simulink model "GFLIB_ControllerPIr_BAM_F32"  (Simulink 7.3)
settings: Solver=ode45  StartTime=0.0  StopTime=10.0  RelTol=1e-3
undefined symbols (not defined in the file): f32CC1, f32CC2, u16NShift
settings Model: Creator=RE004C  LastModifiedBy=RE004C
settings HardwareCC: ProdIntDivRoundTo=Zero  ProdEndianess=BigEndian  ProdHWDeviceType=Freescale->32-bit PowerPC

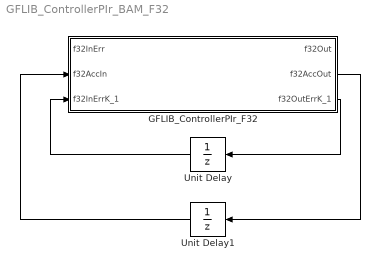
== system GFLIB_ControllerPIr_BAM_F32 ==
  GFLIB_ControllerPIr_F32 : Subsystem  mask(GFLIB_ControllerPIr_F32){f32CC1=f32CC1, f32CC2=f32CC2, u16NShift=u16NShift}
      mask help: Bit accurate model of reccurent form PI controller. All parameters as well as input and output are 32-bit integers except for u16NShift parameter which is 16-bit unsigned integer.
      mask init:
      | pos = get_param(gcb, 'Position');width = pos(3) - pos(1); height = pos(4) - pos(2);tX=width/2;tY=height*0.9;
      mask Display:
      | color('black');
      | port_label('input',1,'f32InErr');
      | port_label('input',2,'f32AccIn');
      | port_label('input',3,'f32InErrK_1');
      | port_label('output',1,'f32Out');
      | port_label('output',2,'f32AccOut');
      | port_label('output',3,'f32OutErrK_1');
      | color('black');
      | disp('GFLIB_ControllerPIr_F32');
      | color('blue');
      | text(tX,tY, 'BAM', 'horizontalAlignment', 'center');
  Unit Delay : UnitDelay  SampleTime=-1
  Unit Delay1 : UnitDelay  SampleTime=-1
  wires:
  GFLIB_ControllerPIr_F32/3(f32OutErrK_1) -> Unit Delay/1
  Unit Delay/1 -> GFLIB_ControllerPIr_F32/3(f32InErrK_1)
  GFLIB_ControllerPIr_F32/2(f32AccOut) -> Unit Delay1/1
  Unit Delay1/1 -> GFLIB_ControllerPIr_F32/2(f32AccIn)

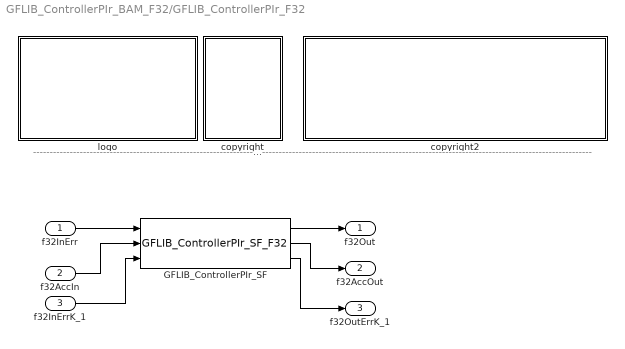
== system GFLIB_ControllerPIr_BAM_F32/GFLIB_ControllerPIr_F32 ==
  note: ---------------------------------------------------------------------------------------------------------------------------------------------------------------------------------------------------
  f32InErr : Inport  OutDataType=fixdt(1, 16)  OutScaling=2^0
  f32AccIn : Inport  Port=2  OutDataType=fixdt(1, 16)  OutScaling=2^0
  f32InErrK_1 : Inport  Port=3  OutDataType=fixdt(1, 16)  OutScaling=2^0
  GFLIB_ControllerPIr_SF : S-Function  FunctionName=GFLIB_ControllerPIr_SF_F32  Parameters=f32CC1,f32CC2,u16NShift  EnableBusSupport=off
  copyright : Subsystem
      mask Display: text(10,90,'FILE:');text(10,75,'DESRIPTION:')text(10,60,'COPYRIGHT:')text(10,45,'VERSION:')text(10,30,'DATE:')
  copyright2 : Subsystem
      mask Display: text(10,90,'GFLIB_ControllerPIr_BAM_F32.mdl');text(10,75,'Recurrent form of a standard PI controller without implemented anti-windup.');text(10,60,'Freescale')text(10,45,'0.1');text(10,30,'20-Jan-2012');
  logo : Subsystem
      mask Display: image(imread('logo.jpg'))
  f32Out : Outport  OutDataType=fixdt(1, 16)  OutScaling=2^0
  f32AccOut : Outport  Port=2  OutDataType=fixdt(1, 16)  OutScaling=2^0
  f32OutErrK_1 : Outport  Port=3  OutDataType=fixdt(1, 16)  OutScaling=2^0
  wires:
  f32InErr/1 -> GFLIB_ControllerPIr_SF/1
  GFLIB_ControllerPIr_SF/1 -> f32Out/1
  f32AccIn/1 -> GFLIB_ControllerPIr_SF/2
  f32InErrK_1/1 -> GFLIB_ControllerPIr_SF/3
  GFLIB_ControllerPIr_SF/2 -> f32AccOut/1
  GFLIB_ControllerPIr_SF/3 -> f32OutErrK_1/1

== system GFLIB_ControllerPIr_BAM_F32/GFLIB_ControllerPIr_F32/copyright ==

== system GFLIB_ControllerPIr_BAM_F32/GFLIB_ControllerPIr_F32/copyright2 ==

== system GFLIB_ControllerPIr_BAM_F32/GFLIB_ControllerPIr_F32/logo ==
